simulink model "Sample_v_0_1"  (R2021b)
settings: Solver=VariableStepAuto  StartTime=0.0  StopTime=10.0  RelTol=1e-3
values from neighbouring files (symbols this model uses):
  KeyOff = 0    [Sample_v_0_1_Parameter.m]
  Two = 2    [Sample_v_0_1_Parameter.m]
undefined symbols (not defined in the file or in its folder): Four_bb, SystemOn
settings Model: Creator=ygkwon  LastModifiedBy=ygkwon

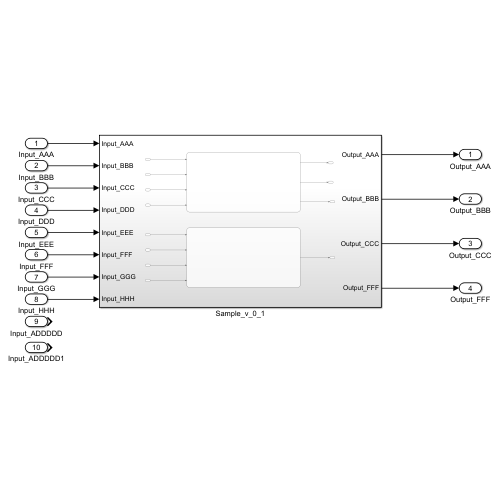
[thumbnail: Simulink's stored preview of the top-level diagram]
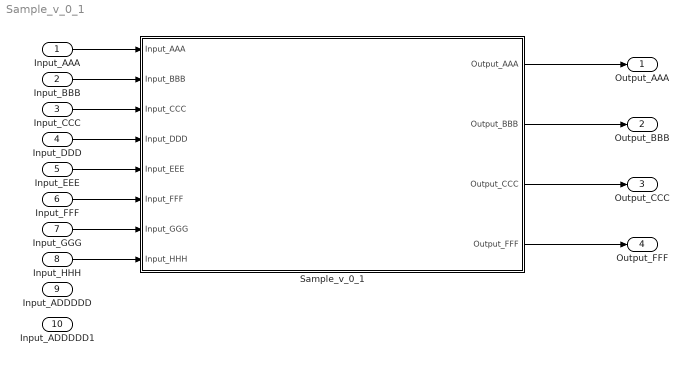
== system Sample_v_0_1 ==
  Input_AAA : Inport
  Input_BBB : Inport  Port=2
  Input_CCC : Inport  Port=3
  Input_DDD : Inport  Port=4
  Input_EEE : Inport  Port=5
  Input_FFF : Inport  Port=6
  Input_GGG : Inport  Port=7
  Input_HHH : Inport  Port=8
  Input_ADDDDD : Inport  Port=9
  Input_ADDDDD1 : Inport  Port=10
  Sample_v_0_1 : Subsystem
  Output_AAA : Outport
  Output_BBB : Outport  Port=2
  Output_CCC : Outport  Port=3
  Output_FFF : Outport  Port=4
  wires:
  Input_AAA/1 -> Sample_v_0_1/1(Input_AAA)
  Input_BBB/1 -> Sample_v_0_1/2(Input_BBB)
  Input_CCC/1 -> Sample_v_0_1/3(Input_CCC)
  Input_DDD/1 -> Sample_v_0_1/4(Input_DDD)
  Sample_v_0_1/1(Output_AAA) -> Output_AAA/1
  Sample_v_0_1/2(Output_BBB) -> Output_BBB/1
  Sample_v_0_1/3(Output_CCC) -> Output_CCC/1
  Input_EEE/1 -> Sample_v_0_1/5(Input_EEE)
  Input_FFF/1 -> Sample_v_0_1/6(Input_FFF)
  Input_GGG/1 -> Sample_v_0_1/7(Input_GGG)
  Input_HHH/1 -> Sample_v_0_1/8(Input_HHH)
  Sample_v_0_1/4(Output_FFF) -> Output_FFF/1

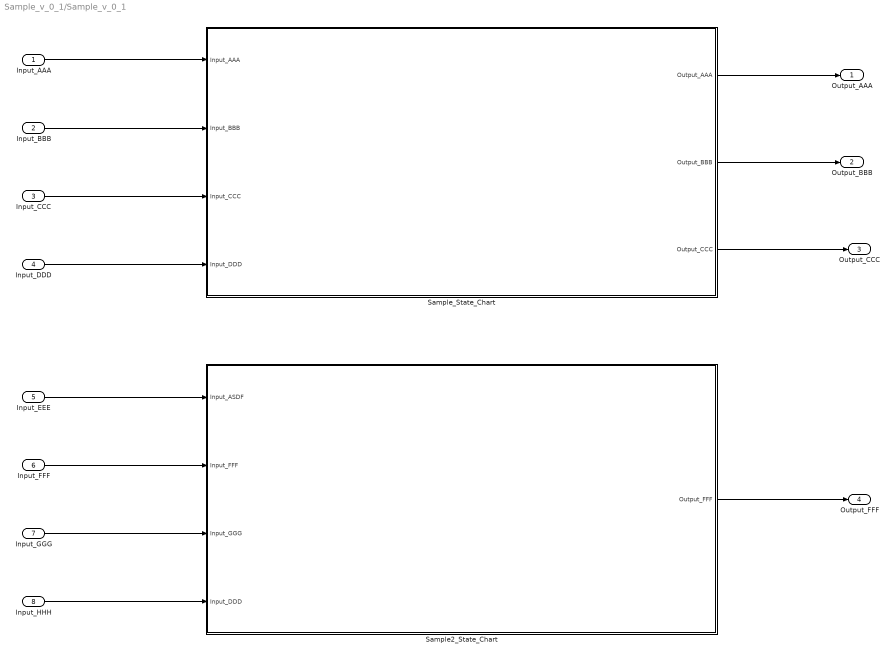
== system Sample_v_0_1/Sample_v_0_1 ==
  Input_AAA : Inport
  Input_BBB : Inport  Port=2
  Input_CCC : Inport  Port=3
  Input_DDD : Inport  Port=4
  Input_EEE : Inport  Port=5
  Input_FFF : Inport  Port=6
  Input_GGG : Inport  Port=7
  Input_HHH : Inport  Port=8
  Sample2_State_Chart : Stateflow chart  TreatAsAtomicUnit=on
  Sample_State_Chart : Stateflow chart  TreatAsAtomicUnit=on
  Output_AAA : Outport
  Output_BBB : Outport  Port=2
  Output_CCC : Outport  Port=3
  Output_FFF : Outport  Port=4
  wires:
  Input_BBB/1 -> Sample_State_Chart/2(Input_BBB)
  Input_CCC/1 -> Sample_State_Chart/3(Input_CCC)
  Input_DDD/1 -> Sample_State_Chart/4(Input_DDD)
  Sample_State_Chart/1(Output_AAA) -> Output_AAA/1
  Sample_State_Chart/2(Output_BBB) -> Output_BBB/1
  Sample_State_Chart/3(Output_CCC) -> Output_CCC/1
  Input_EEE/1 -> Sample2_State_Chart/1(Input_ASDF)
  Input_FFF/1 -> Sample2_State_Chart/2(Input_FFF)
  Input_GGG/1 -> Sample2_State_Chart/3(Input_GGG)
  Input_HHH/1 -> Sample2_State_Chart/4(Input_DDD)
  Sample2_State_Chart/1(Output_FFF) -> Output_FFF/1
  Input_AAA/1 -> Sample_State_Chart/1(Input_AAA)

== stateflow chart Sample_v_0_1/Sample2_State_Chart ==
  state Sample2_State_Chart
    state Stop
      en:
      Output_FFF = Four_bb;
    state Start
      Output_FFF = Two;
    (default) -> Stop
    Stop -> Start : [Input_EEE==SystemOn]
    Start -> Stop : [Input_EEE==KeyOff]
  (default) -> Sample2_State_Chart
  data: Input_ASDF input uint8; Input_FFF input uint8; Input_GGG input uint8; Input_DDD input uint8; Output_FFF output uint8; Four_bb parameter uint8; Two parameter uint8; SystemOn parameter uint8; KeyOff parameter uint8

== stateflow chart Sample_v_0_1/Sample_State_Chart ==
  state Sample_State_Chart
    state Stop
      en:
      Output_AAA = Four_bb;
      b_Running = Off;
    state Start
      Output_AAA = Two;
      b_Running = On;
    (default) -> Stop
    Stop -> Start : [Input_AAA==SystemOn]
    Start -> Stop : [Input_AAA==Four_bb]
  state Test_for [function]
    (default) -> (junction 28)
    (junction 28) -> (junction 32) [order 2] : [Input_CCC == Four_bb]
    (junction 28) -> (junction 30) [order 1]
    (junction 32) -> (junction 33)
    (junction 33) -> (junction 30)
    (junction 30) -> (junction 37)
  (default) -> Sample_State_Chart
  data: Input_AAA input uint8; Input_BBB input uint8; Input_CCC input uint8; Input_DDD input uint8; Output_AAA output uint8; Output_BBB output uint8; Output_CCC output uint8; Four_bb parameter uint8; Two parameter uint8; SystemOn parameter uint8; KeyOff parameter uint8; b_Running local boolean; On parameter boolean; Off parameter boolean
